simulink model "simulator"  (R2022b)
settings: Solver=FixedStepAuto  StartTime=0.0  StopTime=1800  FixedStep=1/7000  RelTol=1e-7
undefined symbols (not defined in the file): simdb
libraries: sim_lib x40, simulink_extras x15, matrix_library x9, simulink x1
(part 3 of 3)

== system simulator/Plant/Forces & Moments/Aerodynamics/Aerodynamic Coefficients/Sideforce Coefficient ==
  In Bus Element : Inport  PortName=params  Element=M
  In Bus Element1 : Inport  PortName=params  Element=AoA
  In Bus Element2 : Inport  PortName=params  Element=delta_el
  In Bus Element3 : Inport  PortName=params  Element=delta_er
  In Bus Element4 : Inport  PortName=params  Element=delta_rl
  In Bus Element5 : Inport  PortName=params  Element=AoS
  In Bus Element6 : Inport  PortName=params  Element=delta_rr
  Add : Sum  Inputs=+-+-
  Add2 : Sum
  Add3 : Sum  Inputs=+++
  CSb0 : Interpolation_n-D  Table=simdb.aero.CSb0  RequireIndexFractionAsBus=on  RemoveProtectionIndex=on  InternalRulePriority=Speed
      settings: InputPortMap=u0,u1
  CSbel : Interpolation_n-D  NumberOfTableDimensions=3  Table=simdb.aero.CSbel  RequireIndexFractionAsBus=on  RemoveProtectionIndex=on  InternalRulePriority=Speed
      settings: InputPortMap=u0,u1,u2
  CSber : Interpolation_n-D  NumberOfTableDimensions=3  Table=simdb.aero.CSbel  RequireIndexFractionAsBus=on  RemoveProtectionIndex=on  InternalRulePriority=Speed
      settings: InputPortMap=u0,u1,u2
  CSel : Interpolation_n-D  NumberOfTableDimensions=3  Table=simdb.aero.CSel  RequireIndexFractionAsBus=on  RemoveProtectionIndex=on  InternalRulePriority=Speed
      settings: InputPortMap=u0,u1,u2
  CSer : Interpolation_n-D  NumberOfTableDimensions=3  Table=simdb.aero.CSel  RequireIndexFractionAsBus=on  RemoveProtectionIndex=on  InternalRulePriority=Speed
      settings: InputPortMap=u0,u1,u2
  CSrl : Interpolation_n-D  NumberOfTableDimensions=3  Table=simdb.aero.CSrl  RequireIndexFractionAsBus=on  RemoveProtectionIndex=on  InternalRulePriority=Speed
      settings: InputPortMap=u0,u1,u2
  CSrr : Interpolation_n-D  NumberOfTableDimensions=3  Table=simdb.aero.CSrl  RequireIndexFractionAsBus=on  RemoveProtectionIndex=on  InternalRulePriority=Speed
      settings: InputPortMap=u0,u1,u2
  Product1 : Product
  CS : Outport
  wires:
  In Bus Element1/1 -> CSrr/1, CSrl/1, CSer/1, CSel/1, CSber/1, CSbel/1, CSb0/1
  In Bus Element/1 -> CSrr/3, CSrl/3, CSer/3, CSel/3, CSber/3, CSbel/3, CSb0/2
  CSbel/1 -> Add3/2
  CSber/1 -> Add3/3
  CSb0/1 -> Add3/1
  Add3/1 -> Product1/2
  In Bus Element5/1 -> Product1/1
  In Bus Element2/1 -> CSel/2, CSbel/2
  In Bus Element3/1 -> CSer/2, CSber/2
  In Bus Element6/1 -> CSrr/2
  In Bus Element4/1 -> CSrl/2
  CSer/1 -> Add/2
  CSrl/1 -> Add/3
  CSel/1 -> Add/1
  CSrr/1 -> Add/4
  Add2/1 -> CS/1
  Add/1 -> Add2/2
  Product1/1 -> Add2/1

== system simulator/Plant/Forces & Moments/Aerodynamics/Aerodynamic Coefficients/Yaw Moment Coefficient ==
  In Bus Element : Inport  PortName=params  Element=M
  In Bus Element1 : Inport  PortName=params  Element=AoA
  In Bus Element2 : Inport  PortName=params  Element=delta_el
  In Bus Element3 : Inport  PortName=params  Element=delta_er
  In Bus Element4 : Inport  PortName=params  Element=delta_rl
  In Bus Element5 : Inport  PortName=params  Element=AoS
  In Bus Element6 : Inport  PortName=params  Element=delta_rr
  Add2 : Sum
  Add3 : Sum  Inputs=+++
  Add4 : Sum  Inputs=+-+-
  Cnb0 : Interpolation_n-D  Table=simdb.aero.Cnb0  RequireIndexFractionAsBus=on  RemoveProtectionIndex=on  InternalRulePriority=Speed
      settings: InputPortMap=u0,u1
  Cnbrl : Interpolation_n-D  NumberOfTableDimensions=3  Table=simdb.aero.Cnbrl  RequireIndexFractionAsBus=on  RemoveProtectionIndex=on  InternalRulePriority=Speed
      settings: InputPortMap=u0,u1,u2
  Cnbrr : Interpolation_n-D  NumberOfTableDimensions=3  Table=simdb.aero.Cnbrl  RequireIndexFractionAsBus=on  RemoveProtectionIndex=on  InternalRulePriority=Speed
      settings: InputPortMap=u0,u1,u2
  Cnel : Interpolation_n-D  NumberOfTableDimensions=3  Table=simdb.aero.Cnel  RequireIndexFractionAsBus=on  RemoveProtectionIndex=on  InternalRulePriority=Speed
      settings: InputPortMap=u0,u1,u2
  Cner : Interpolation_n-D  NumberOfTableDimensions=3  Table=simdb.aero.Cnel  RequireIndexFractionAsBus=on  RemoveProtectionIndex=on  InternalRulePriority=Speed
      settings: InputPortMap=u0,u1,u2
  Cnrl : Interpolation_n-D  NumberOfTableDimensions=3  Table=simdb.aero.Cnrl  RequireIndexFractionAsBus=on  RemoveProtectionIndex=on  InternalRulePriority=Speed
      settings: InputPortMap=u0,u1,u2
  Cnrr : Interpolation_n-D  NumberOfTableDimensions=3  Table=simdb.aero.Cnrl  RequireIndexFractionAsBus=on  RemoveProtectionIndex=on  InternalRulePriority=Speed
      settings: InputPortMap=u0,u1,u2
  Product1 : Product
  Cn : Outport
  wires:
  Add2/1 -> Cn/1
  In Bus Element1/1 -> Cner/1, Cnel/1, Cnrr/1, Cnrl/1, Cnbrr/1, Cnbrl/1, Cnb0/1
  In Bus Element4/1 -> Cnrl/2, Cnbrl/2
  In Bus Element6/1 -> Cnrr/2, Cnbrr/2
  In Bus Element3/1 -> Cner/2
  In Bus Element2/1 -> Cnel/2
  In Bus Element/1 -> Cnbrl/3, Cner/3, Cnel/3, Cnrr/3, Cnrl/3, Cnbrr/3, Cnb0/2
  Cnbrl/1 -> Add3/2
  Cnb0/1 -> Add3/1
  Cnbrr/1 -> Add3/3
  Add3/1 -> Product1/2
  In Bus Element5/1 -> Product1/1
  Cnrr/1 -> Add4/2
  Cnel/1 -> Add4/3
  Cner/1 -> Add4/4
  Cnrl/1 -> Add4/1
  Add4/1 -> Add2/2
  Product1/1 -> Add2/1

== matlab function simulator/Control System/Longitudinal Controller SS Model ==
  data: x input; A output; B output; coeff_deriv input; rho input; S parameter; c parameter; Iyy parameter; m parameter
function [A, B] = fcn(x, coeff_deriv, rho, S, c, Iyy, m)
    A = zeros(2,2);
    B = zeros(2,1);

    qdyn = 0.5*rho*x(4)^2;

    dCL_dAoA = coeff_deriv(1) * 180/pi;
    dCm_dAoA = coeff_deriv(2) * 180/pi;
    dCm_de = coeff_deriv(3);

    A(1,2) = qdyn*S*c/Iyy * dCm_dAoA;
    A(2,1) = 1;
    A(2,2) = -qdyn*S/(m*x(4)) * dCL_dAoA * cos(x(12))^2;
    %A(3,2) = -1;

    %B(1,1) = qdyn*S*c/Iyy * dCm_de;
    B(1,1) = 1/Iyy;
end

== matlab function simulator/Control System/Lateral Controller SS Model ==
  data: x input; CL input; A output; B output; coeff_deriv input; rho input; S parameter; b parameter; Ixx parameter; Izz parameter; m parameter; mu parameter
function [A, B] = fcn(x, CL, coeff_deriv, rho, S, b, Ixx, Izz, m, mu)
    A = zeros(4,4);
    B = zeros(4,4);

    cg = cos(x(5));
    tg = tan(x(5));
    sa = sin(x(10));
    ca = cos(x(10));
    cs = cos(x(12));

    qdyn = 0.5*rho*x(4)^2;
    g = mu/x(1)^2;
    L = qdyn*CL*S;

    dCl_dAoS    = coeff_deriv(4) * 180/pi;
    dCl_da      = coeff_deriv(5);
    dCn_dAoS    = coeff_deriv(6) * 180/pi;
    dCn_da      = coeff_deriv(7);
    dCn_dr      = coeff_deriv(8);
    
    A(1,3) = qdyn*S*b/Ixx * dCl_dAoS;
    A(2,3) = qdyn*S*b/Izz * dCn_dAoS;
    A(3,1) = sa;
    A(3,2) = -ca;
    A(3,4) = (x(4)/x(1) - g/x(4))*cg*cs;
    A(4,1) = -ca;
    A(4,2) = -sa;
    A(4,3) = -(L/(m*x(4))*cs + (x(4)/x(1) - g/x(4))*cg)*cs;
    A(4,4) = L/(m*x(4))*tg*cs;

    B(1,1) = qdyn*S*b/Ixx * dCl_da;
    B(1,3) = 1/Ixx;
    B(2,1) = qdyn*S*b/Izz * dCn_da;
    B(2,2) = qdyn*S*b/Izz * dCn_dr;
    B(2,4) = 1/Izz;
end

== matlab function simulator/Guidance System/Longitudinal Guidance SS Model ==
  data: x input; u input; coeffs input; A output; B output; rho input; drho_dR input; mu parameter; m parameter; S parameter
function [A, B] = fcn(x, u, coeffs, rho, drho_dR, mu, m, S)
    A = zeros(3);
    B = zeros(3, 2);

    sg = sin(x(5));
    cg = cos(x(5));

    ss = sin(u(1));
    cs = cos(u(1));

    CD = coeffs(1);
    CL = coeffs(2);
    dCD_dAoA = coeffs(3) * 180/pi;
    dCL_dAoA = coeffs(4) * 180/pi;

    g = mu/x(1)^2;

    A(1,2) = sg;
    A(1,3) = x(4)*cg;

    A(2,1) = -x(4)^2*CD*S/(2*m)*drho_dR + 2*g/x(1)*sg;
    A(2,2) = -rho*x(4)*CD*S/m;
    A(2,3) = -g*cg;

    A(3,1) = x(4)*CL*S/(2*m)*drho_dR*cs + g*(2/(x(1)*x(4)) - x(4)/mu)*cg;
    A(3,2) = rho*CL*S/(2*m)*cs + (1/x(1) + g/x(4)^2)*cg;
    A(3,3) = -(x(4)/x(1) - g/x(4))*sg;

    B(2,1) = -rho*x(4)^2*S/(2*m)*dCD_dAoA;
    B(3,1) = rho*x(4)*S/(2*m)*dCL_dAoA*cs;
    B(3,2) = -rho*x(4)*CL*S/(2*m)*ss;
end

% function [A, B] = fcn(x, u, CD, CL, rho, drho_dR, mu, m, S)
%     x
%     A = zeros(6);
%     B = zeros(6, 1);
% 
%     sd = sin(x(3));
%     cd = cos(x(3));
%     td = tan(x(3));
%     sg = sin(x(5));
%     cg = cos(x(5));
%     sc = sin(x(6));
%     cc = cos(x(6));
% 
%     ss = sin(u(1));
%     cs = cos(u(1));
% 
%     g = mu/x(1)^2;
% 
%     A(1,4) = sg;
%     A(1,5) = x(4)*cg;
% 
%     A(2,1) = -x(4)*sc*cg/(x(1)^2*cd);
%     A(2,3) = x(4)*sc*cg*sd/(x(1)*cd^2);
%     A(2,4) = sc*cg/(x(1)*cd);
%     A(2,5) = -x(4)*sc*sg/(x(1)*cd);
%     A(2,6) = x(4)*cc*cg/(x(1)*cd);
% 
%     A(3,1) = -x(4)*cc*cg/(x(1)^2);
%     A(3,4) = cc*cg/x(1);
%     A(3,5) = -x(4)*cc*sg/x(1);
%     A(3,6) = -x(4)*sc*cg/x(1);
% 
%     A(4,1) = -x(4)^2*CD*S/(2*m)*drho_dR;
%     A(4,4) = -rho*x(4)*CD*S/m - g*sg;
%     A(4,5) = -g*cg;
% 
%     A(5,1) = x(4)*CL*S/(2*m)*drho_dR*cs - g*(x(4)/mu + 2/(x(1)*x(4)))*cg;
%     A(5,4) = rho*CL*S/(2*m)*cs + (1/x(1) + g/x(4)^2)*cg;
%     A(5,5) = -(x(4)/x(1) - g/x(4))*sg;
% 
%     A(6,1) = -x(4)*CL*S/(2*m)*drho_dR*ss/cg - x(4)/(x(1)^2)*cg*td*sc;
%     A(6,3) = x(4)/x(1)*cg*sc/(cd^2);
%     A(6,4) = -rho*CL*S/(2*m)*ss/cg + cg*td*sc/x(1);
%     A(6,5) = -rho*x(4)*CL*S/(2*m)*sg*ss/(cg^2) - x(4)*sg*td*sc/x(1);
%     A(6,6) = x(4)*cg*td*cc/x(1);
% 
%     B(5,1) = -rho*x(4)*CL*S/(2*m)*ss;
%     B(6,1) = -rho*x(4)*CL*S/(2*m)*cs/cg;
% end

== matlab function simulator/Plant/DKE ==
  data: x input; dy output; F_RCS input; F_ae input; F_g input; M_RCS input; M_ae input; m parameter; omega_cb parameter; I parameter
function dy = fcn(x, F_RCS, F_ae, F_g, M_RCS, M_ae, m, omega_cb, I)

%% Trigonometric angle definitions
% Latitude Coordinate (delta)
sd = sin(x(3));
cd = cos(x(3));
td = tan(x(3));

% Glideslope Angle (gamma)
sg = sin(x(5));
cg = cos(x(5));

% Heading Angle (chi)
sc = sin(x(6));
cc = cos(x(6));

% Angle of Attack, Groundspeed-based (alpha)
sa = sin(x(10));
ca = cos(x(10));

% Sideslip Angle, Groundspeed-based (alpha)
sb = sin(x(11));
cb = cos(x(11));

% Banking Angle, Groundspeed-based (alpha)
ss = sin(x(12));
cs = cos(x(12));

%% Derive Forces in Vertical Frame
F = F_RCS + F_g + F_ae;
F = [F(1); -F(3); F(2)];

%% Derive Moments in Body Frame
M = M_RCS + M_ae;

dy = zeros(size(x));

%% Translational Kinematics
dy(1) = x(4)*sg;
dy(2) = x(4)*sc*cg / (x(1)*cd);
dy(3) = x(4)*cc*cg / x(1);

%% Translational Dynamics
dy(4) = F(1)/m + omega_cb^2*x(1)*cd * (sg*cd - cg*sd*cc);
dy(5) = (F(2)/m + 2*omega_cb*x(4)*cd*sc + x(4)^2/x(1)*cg + ...
   omega_cb^2*x(1)*cd * (cd*cg + sg*sd*cc)) / x(4);
dy(6) = (F(3)/m + 2*omega_cb*x(4) * (sd*cg - cd*sg*cc) + ...
   x(4)^2/x(1)*cg^2*td*sc + omega_cb^2*x(1)*cd*sd*sc) / (x(4)*cg);

% dy(1) = x(4)*sg;
% dy(2) = x(4)*sc*cg / (x(1)*cd);
% dy(3) = x(4)*cc*cg / x(1);
% dy(4) = F(1)/m + omega_cb^2*x(1)*cd*(sg*cd - cg*sd*cc);
% dy(5) = (F(2)/m + 2*omega_cb*x(4)*cd*sc + x(4)^2/x(1)*cg + ...
%     omega_cb^2*x(1)*cd*(cd*cg + sg*sd*cc)) / x(4);
% dy(6) = (F(3)/m + 2*omega_cb*x(4)*(sd*cg - cd*sg*cc) + ...
%     x(4)^2/x(1)*cg^2*td*sc + omega_cb^2*x(1)*cd*sd*sc)/(x(4)*cg);

%% Rotational Dynamics
dy(7:9) = inv(I) * (M - cross(x(7:9), I*x(7:9)));
dy(7) = 0; dy(9) = 0;
%dy(7:9) = [0;0;0];

%% Groundspeed-based Aerodynamic Angles
dy(10) = (-x(7)*ca*sb + x(8)*cb - x(9)*sa*sb + ss*(dy(6)*cg - ...
   dy(3)*sc*sg + (dy(2) + omega_cb) * (cd*cc*sg - sd*cg)) - ...
   cs*(dy(5) - dy(3)*cc - (dy(2) + omega_cb) * cd*sc)) / cb;
% 
% dy(11) = x(7)*sa - x(9)*ca + ss*(dy(5) - dy(3)*cc - ...
%    (dy(2) + omega_cb) * cd*sc) + cs*(dy(6)*cg - dy(3)*sc*sg + ...
%    (dy(2) + omega_cb) * (cd*cc*sg - sd*cg));
% 
% dy(12) = -x(7)*ca*cb - x(8)*sb - x(9)*sa*cb + dy(10)*sb - dy(6)*sg - ...
%     dy(3)*sc*cg + (dy(2) + omega_cb) * (cd*cc*cg + sd*sg);
%dy(10:12) = [0; 0; 0];

%% Rotational Kinematics
dy(13:16) = -0.5 * quatmul([0; x(7:9)], x(13:16));

== matlab function simulator/Guidance System/Reference Trajectory/Ref Angle of Attack ==
  data: M input; AoA output
function AoA = fcn(M)
    f = deg2rad(15);
    g = deg2rad(40);
    
    K = 1;
    M_c = 7;

    s = (1 + tanh(K.*(M - M_c))) ./ 2;
    AoA = g.*s + (1-s).*f;
end

== matlab function simulator/Navigation System/MATLAB Function ==
  data: x input; dx output; y input; mu parameter; K parameter
function dx = fcn(x, y, mu, K)
    dx = zeros(22,1);
    
    R = norm(x(1:3));
    eps = 1 - (x(13)^2 + x(14)^2 + x(15)^2 + x(16)^2);


    dx(1:3) = x(4:6);
    dx(4:6) = quatrot(x(13:16), y(1:3)) - mu/R^3*x(1:3);
    dx(13:16) = 0.5*quatmul([0; y(4:6)], x(13:16)) + K*eps*x(13:16);
end

== matlab function simulator/Navigation System/Extended Kalman Filter/estimation function ==
  data: x input; x_est output; dt input; mu parameter; K parameter
function x_est = fcn(x, dt, mu, K)
    x_est = zeros(size(x));

    g = -mu/norm(x(1:3))^3 * x(1:3);
    eps = 1 - (x(13)^2 + x(14)^2 + x(15)^2 + x(16)^2);

    x_est(1:3) = x(1:3) + x(4:6)*dt + 0.5*(x(7:9) + g)*dt^2;
    x_est(4:6) = x(4:6) + (x(7:9) + g)*dt;
    x_est(7:9) = x(7:9);
    x_est(10:12) = x(10:12);
    x_est(13:16) = x(13:16) + (0.5*quatmul([0; x(10:12)], x(13:16)) + K*eps*x(13:16))*dt;
    x_est(17:19) = x(17:19);
    x_est(20:22) = x(20:22);
end

== matlab function simulator/Navigation System/Extended Kalman Filter/observation function ==
  data: x input; z output; dt input; Ma parameter; Mo parameter
function z = fcn(x, dt, Ma, Mo)
    z = zeros(6,1);
    I = eye(3);

    z(1:3) = ((I + Ma)*quatrot(quatconj(x(13:16)), x(7:9)) + x(17:19))*dt;
    z(4:6) = ((I + Mo)*x(10:12) + x(20:22))*dt;
end

== matlab function simulator/Navigation System/Extended Kalman Filter/estimation matrix ==
  data: x input; F output; mu parameter
function F = fcn(x, mu)
    F = zeros(22);

    R = norm(x(1:3));
    I = eye(3);
    dg = mu/R^5*(3*x(1:3)*x(1:3)' - R^2*I);

    dq_dw = 0.5*[-x(14) -x(15) -x(16);
                  x(13)  x(16) -x(15);
                 -x(16)  x(13)  x(14);
                  x(15) -x(14)  x(13)];

    Omega = [   0  -x(10) -x(11) -x(12);
             x(10)     0  -x(12)  x(11);
             x(11)  x(12)     0  -x(10);
             x(12) -x(11)  x(10)     0];

    F(1:3,4:6) = I;

    F(4:6,1:3) = dg;
    F(4:6,7:9) = I;

    F(13:16,10:12) = dq_dw;
    F(13:16,13:16) = 0.5*Omega;
end

== matlab function simulator/Navigation System/Extended Kalman Filter/observation matrix ==
  data: x input; H output; dt input; Ma parameter; Mo parameter
function H = fcn(x, dt, Ma, Mo)
    H = zeros(6,22);
    
    I = eye(3);

    H(1:3,7:9) = (I + Ma) * [    1 - 2*(x(15)^2 + x(16)^2)       2*(x(14)*x(15) + x(13)*x(16))       2*(x(14)*x(16) - x(13)*x(15));
                             2*(x(14)*x(15) - x(13)*x(16))           1 - 2*(x(14)^2 + x(16)^2)       2*(x(15)*x(16) + x(13)*x(14));
                             2*(x(14)*x(16) + x(13)*x(15))       2*(x(15)*x(16) - x(13)*x(14))           1 - 2*(x(14)^2 + x(15)^2)] * dt;

    qw_x = x(13)*x(7);  qw_y = x(13)*x(8);  qw_z = x(13)*x(9);
    qx_x = x(14)*x(7);  qx_y = x(14)*x(8);  qx_z = x(14)*x(9);
    qy_x = x(15)*x(7);  qy_y = x(15)*x(8);  qy_z = x(15)*x(9);
    qz_x = x(16)*x(7);  qz_y = x(16)*x(8);  qz_z = x(16)*x(9);
    
    H(1:3,13:16) = 2*(I + Ma) * [ qz_y - qy_z             qy_y + qz_z    -2*qy_x + qx_y - qw_z    -2*qz_x + qw_y + qx_z;
                                 -qz_x + qx_z    qy_x - 2*qx_y + qw_z              qx_x + qz_z    -qw_x - 2*qz_y + qy_z;
                                  qy_x - qx_y    qz_x - qw_y - 2*qx_z     qw_x + qz_y - 2*qy_z              qx_x + qy_y] * dt;
    H(1:3,17:19) = I*dt;

    H(4:6,10:12) = (I + Mo)*dt;
    H(4:6,20:22) = I*dt;
end
